simulink model "Intergration_simu"  (R2018b)
settings: Solver=FixedStepDiscrete  StartTime=0.0  StopTime=14  FixedStep=0.005  RelTol=1e-3
PostLoadFcn:
  | if any(exist('dsrtsu_mdlpostloadfcn', 'file') ~= 0), dsrtsu_mdlpostloadfcn('Execute', bdroot); end
values from neighbouring files (symbols this model uses):
  P_x165_On = 1.0    [CAN_Tx.sldd]
  P_x242_On = 1.0    [CAN_Tx.sldd]
  P_x246_On = 1.0    [CAN_Tx.sldd]
libraries: rtican x112, simulink x59
(part 31 of 31)

== system Intergration_simu/TX/ESC_FrontWheelSpeedKPH_0x123/Subsystem ==
  <WhlGndVelLDrvn_Radar> : Inport
  Bitwise Operator1 : simulink/Logic and Bit Operations/Bitwise Operator  logicop=AND  UseBitMask=on  BitMask=bin2dec('11111111')  BitMaskRealWorld=Stored Integer
  Constant : Constant  Value=0.05625
  Constant1 : Constant  Value=0.05625
  Data Type Conversion1 : DataTypeConversion  OutDataTypeStr=uint16
  Data Type Conversion2 : DataTypeConversion  OutDataTypeStr=uint8
  Divide : Product  Inputs=*/
  Multiply : Product
  Shift Arithmetic1 : ArithShift  BitShiftNumber=5  BitShiftDirection=Right
  Out1 : Outport
  Byte0 : Outport  Port=2
  Output : Outport  Port=3
  wires:
  Bitwise Operator1/1 -> Data Type Conversion2/1
  Shift Arithmetic1/1 -> Bitwise Operator1/1
  Divide/1 -> Data Type Conversion1/1
  Constant/1 -> Divide/2
  Constant1/1 -> Multiply/1
  Data Type Conversion1/1 -> Output/1, Multiply/2, Shift Arithmetic1/1
  <WhlGndVelLDrvn_Radar>/1 -> Divide/1
  Multiply/1 -> Out1/1
  Data Type Conversion2/1 -> Byte0/1

== system Intergration_simu/TX/ESC_FrontWheelSpeedKPH_0x123/Subsystem1 ==
  In1 : Inport
  <LDrvnWhlRotlDircn> : Inport  Port=2
  Add : Sum
  Bitwise Operator1 : simulink/Logic and Bit Operations/Bitwise Operator  logicop=AND  UseBitMask=on  BitMask=bin2dec('00000110')  BitMaskRealWorld=Stored Integer
  Bitwise Operator2 : simulink/Logic and Bit Operations/Bitwise Operator  logicop=AND  UseBitMask=on  BitMask=bin2dec('11111000')  BitMaskRealWorld=Stored Integer
  Data Type Conversion1 : DataTypeConversion  OutDataTypeStr=uint8
  Data Type Conversion2 : DataTypeConversion  OutDataTypeStr=uint8
  Shift Arithmetic1 : ArithShift  BitShiftNumber=1  BitShiftDirection=Left
  Shift Arithmetic2 : ArithShift  BitShiftNumber=3  BitShiftDirection=Left
  Byte1 : Outport
  wires:
  <LDrvnWhlRotlDircn>/1 -> Data Type Conversion1/1
  Bitwise Operator2/1 -> Data Type Conversion2/1
  Data Type Conversion1/1 -> Shift Arithmetic1/1
  Bitwise Operator1/1 -> Add/1
  Shift Arithmetic1/1 -> Bitwise Operator1/1
  Add/1 -> Byte1/1
  Shift Arithmetic2/1 -> Bitwise Operator2/1
  In1/1 -> Shift Arithmetic2/1
  Data Type Conversion2/1 -> Add/2

== system Intergration_simu/TX/ESC_FrontWheelSpeedKPH_0x123/Subsystem2 ==
  <WhlGndVelLDrvn_Radar> : Inport
  Bitwise Operator1 : simulink/Logic and Bit Operations/Bitwise Operator  logicop=AND  UseBitMask=on  BitMask=bin2dec('11111111')  BitMaskRealWorld=Stored Integer
  Constant : Constant  Value=0.05625
  Constant1 : Constant  Value=0.05625
  Data Type Conversion1 : DataTypeConversion  OutDataTypeStr=uint16
  Data Type Conversion2 : DataTypeConversion  OutDataTypeStr=uint8
  Divide : Product  Inputs=*/
  Multiply : Product
  Shift Arithmetic1 : ArithShift  BitShiftNumber=5  BitShiftDirection=Right
  Out1 : Outport
  Byte2 : Outport  Port=2
  Output : Outport  Port=3
  wires:
  Bitwise Operator1/1 -> Data Type Conversion2/1
  Shift Arithmetic1/1 -> Bitwise Operator1/1
  Divide/1 -> Data Type Conversion1/1
  Constant/1 -> Divide/2
  Constant1/1 -> Multiply/1
  Data Type Conversion1/1 -> Output/1, Multiply/2, Shift Arithmetic1/1
  <WhlGndVelLDrvn_Radar>/1 -> Divide/1
  Multiply/1 -> Out1/1
  Data Type Conversion2/1 -> Byte2/1

== system Intergration_simu/TX/ESC_FrontWheelSpeedKPH_0x123/Subsystem3 ==
  In1 : Inport
  <LDrvnWhlRotlDircn> : Inport  Port=2
  Add : Sum
  Bitwise Operator1 : simulink/Logic and Bit Operations/Bitwise Operator  logicop=AND  UseBitMask=on  BitMask=bin2dec('00000110')  BitMaskRealWorld=Stored Integer
  Bitwise Operator2 : simulink/Logic and Bit Operations/Bitwise Operator  logicop=AND  UseBitMask=on  BitMask=bin2dec('11111000')  BitMaskRealWorld=Stored Integer
  Data Type Conversion1 : DataTypeConversion  OutDataTypeStr=uint8
  Data Type Conversion2 : DataTypeConversion  OutDataTypeStr=uint8
  Shift Arithmetic1 : ArithShift  BitShiftNumber=1  BitShiftDirection=Left
  Shift Arithmetic2 : ArithShift  BitShiftNumber=3  BitShiftDirection=Left
  Byte3 : Outport
  wires:
  <LDrvnWhlRotlDircn>/1 -> Data Type Conversion1/1
  Bitwise Operator2/1 -> Data Type Conversion2/1
  Data Type Conversion1/1 -> Shift Arithmetic1/1
  Bitwise Operator1/1 -> Add/1
  Shift Arithmetic1/1 -> Bitwise Operator1/1
  Add/1 -> Byte3/1
  Shift Arithmetic2/1 -> Bitwise Operator2/1
  In1/1 -> Shift Arithmetic2/1
  Data Type Conversion2/1 -> Add/2

== system Intergration_simu/TX/ESC_FrontWheelSpeedKPH_0x123/Subsystem4 ==
  In1 : Inport
  Bitwise Operator2 : simulink/Logic and Bit Operations/Bitwise Operator  logicop=AND  UseBitMask=on  BitMask=bin2dec('00001111')  BitMaskRealWorld=Stored Integer
  Data Type Conversion1 : DataTypeConversion  OutDataTypeStr=uint8
  Byte6 : Outport
  wires:
  In1/1 -> Data Type Conversion1/1
  Bitwise Operator2/1 -> Byte6/1
  Data Type Conversion1/1 -> Bitwise Operator2/1

== system Intergration_simu/TX/ESC_RearWheelSpeedKPH_0x124/RollingCounter1 ==
  Add2 : Sum
  Constant5 : Constant
  Constant6 : Constant  Value=-1
  Delay : Delay  DelayLength=1
  Switch : Switch  Criteria=u2 > Threshold  Threshold=14
  RC : Outport
  wires:
  Constant6/1 -> Switch/1
  Switch/1 -> Add2/2
  Delay/1 -> RC/1, Switch/3, Switch/2
  Add2/1 -> Delay/1
  Constant5/1 -> Add2/1

== system Intergration_simu/TX/ESC_RearWheelSpeedKPH_0x124/Subsystem ==
  <WhlGndVelLDrvn_Radar> : Inport
  Bitwise Operator1 : simulink/Logic and Bit Operations/Bitwise Operator  logicop=AND  UseBitMask=on  BitMask=bin2dec('11111111')  BitMaskRealWorld=Stored Integer
  Constant : Constant  Value=0.05625
  Constant1 : Constant  Value=0.05625
  Data Type Conversion1 : DataTypeConversion  OutDataTypeStr=uint16
  Data Type Conversion2 : DataTypeConversion  OutDataTypeStr=uint8
  Divide : Product  Inputs=*/
  Multiply : Product
  Shift Arithmetic1 : ArithShift  BitShiftNumber=5  BitShiftDirection=Right
  Out1 : Outport
  Byte0 : Outport  Port=2
  Output : Outport  Port=3
  wires:
  Bitwise Operator1/1 -> Data Type Conversion2/1
  Shift Arithmetic1/1 -> Bitwise Operator1/1
  Divide/1 -> Data Type Conversion1/1
  Constant/1 -> Divide/2
  Constant1/1 -> Multiply/1
  Data Type Conversion1/1 -> Output/1, Multiply/2, Shift Arithmetic1/1
  <WhlGndVelLDrvn_Radar>/1 -> Divide/1
  Multiply/1 -> Out1/1
  Data Type Conversion2/1 -> Byte0/1

== system Intergration_simu/TX/ESC_RearWheelSpeedKPH_0x124/Subsystem1 ==
  In1 : Inport
  <LDrvnWhlRotlDircn> : Inport  Port=2
  Add : Sum
  Bitwise Operator1 : simulink/Logic and Bit Operations/Bitwise Operator  logicop=AND  UseBitMask=on  BitMask=bin2dec('00000110')  BitMaskRealWorld=Stored Integer
  Bitwise Operator2 : simulink/Logic and Bit Operations/Bitwise Operator  logicop=AND  UseBitMask=on  BitMask=bin2dec('11111000')  BitMaskRealWorld=Stored Integer
  Data Type Conversion1 : DataTypeConversion  OutDataTypeStr=uint8
  Data Type Conversion2 : DataTypeConversion  OutDataTypeStr=uint8
  Shift Arithmetic1 : ArithShift  BitShiftNumber=1  BitShiftDirection=Left
  Shift Arithmetic2 : ArithShift  BitShiftNumber=3  BitShiftDirection=Left
  Byte1 : Outport
  wires:
  <LDrvnWhlRotlDircn>/1 -> Data Type Conversion1/1
  Bitwise Operator2/1 -> Data Type Conversion2/1
  Data Type Conversion1/1 -> Shift Arithmetic1/1
  Bitwise Operator1/1 -> Add/1
  Shift Arithmetic1/1 -> Bitwise Operator1/1
  Add/1 -> Byte1/1
  Shift Arithmetic2/1 -> Bitwise Operator2/1
  In1/1 -> Shift Arithmetic2/1
  Data Type Conversion2/1 -> Add/2

== system Intergration_simu/TX/ESC_RearWheelSpeedKPH_0x124/Subsystem2 ==
  <WhlGndVelLDrvn_Radar> : Inport
  Bitwise Operator1 : simulink/Logic and Bit Operations/Bitwise Operator  logicop=AND  UseBitMask=on  BitMask=bin2dec('11111111')  BitMaskRealWorld=Stored Integer
  Constant : Constant  Value=0.05625
  Constant1 : Constant  Value=0.05625
  Data Type Conversion1 : DataTypeConversion  OutDataTypeStr=uint16
  Data Type Conversion2 : DataTypeConversion  OutDataTypeStr=uint8
  Divide : Product  Inputs=*/
  Multiply : Product
  Shift Arithmetic1 : ArithShift  BitShiftNumber=5  BitShiftDirection=Right
  Out1 : Outport
  Byte2 : Outport  Port=2
  Output : Outport  Port=3
  wires:
  Bitwise Operator1/1 -> Data Type Conversion2/1
  Shift Arithmetic1/1 -> Bitwise Operator1/1
  Divide/1 -> Data Type Conversion1/1
  Constant/1 -> Divide/2
  Constant1/1 -> Multiply/1
  Data Type Conversion1/1 -> Output/1, Multiply/2, Shift Arithmetic1/1
  <WhlGndVelLDrvn_Radar>/1 -> Divide/1
  Multiply/1 -> Out1/1
  Data Type Conversion2/1 -> Byte2/1

== system Intergration_simu/TX/ESC_RearWheelSpeedKPH_0x124/Subsystem3 ==
  In1 : Inport
  <LDrvnWhlRotlDircn> : Inport  Port=2
  Add : Sum
  Bitwise Operator1 : simulink/Logic and Bit Operations/Bitwise Operator  logicop=AND  UseBitMask=on  BitMask=bin2dec('00000110')  BitMaskRealWorld=Stored Integer
  Bitwise Operator2 : simulink/Logic and Bit Operations/Bitwise Operator  logicop=AND  UseBitMask=on  BitMask=bin2dec('11111000')  BitMaskRealWorld=Stored Integer
  Data Type Conversion1 : DataTypeConversion  OutDataTypeStr=uint8
  Data Type Conversion2 : DataTypeConversion  OutDataTypeStr=uint8
  Shift Arithmetic1 : ArithShift  BitShiftNumber=1  BitShiftDirection=Left
  Shift Arithmetic2 : ArithShift  BitShiftNumber=3  BitShiftDirection=Left
  Byte3 : Outport
  wires:
  <LDrvnWhlRotlDircn>/1 -> Data Type Conversion1/1
  Bitwise Operator2/1 -> Data Type Conversion2/1
  Data Type Conversion1/1 -> Shift Arithmetic1/1
  Bitwise Operator1/1 -> Add/1
  Shift Arithmetic1/1 -> Bitwise Operator1/1
  Add/1 -> Byte3/1
  Shift Arithmetic2/1 -> Bitwise Operator2/1
  Data Type Conversion2/1 -> Add/2
  In1/1 -> Shift Arithmetic2/1

== system Intergration_simu/TX/ESC_RearWheelSpeedKPH_0x124/Subsystem4 ==
  In1 : Inport
  Bitwise Operator2 : simulink/Logic and Bit Operations/Bitwise Operator  logicop=AND  UseBitMask=on  BitMask=bin2dec('00001111')  BitMaskRealWorld=Stored Integer
  Data Type Conversion1 : DataTypeConversion  OutDataTypeStr=uint8
  Byte6 : Outport
  wires:
  In1/1 -> Data Type Conversion1/1
  Bitwise Operator2/1 -> Byte6/1
  Data Type Conversion1/1 -> Bitwise Operator2/1

== system Intergration_simu/TX/ESC_Status_0x126/RollingCounter1 ==
  Add2 : Sum
  Constant5 : Constant
  Constant6 : Constant  Value=-1
  Delay : Delay  DelayLength=1
  Switch : Switch  Criteria=u2 > Threshold  Threshold=14
  RC : Outport
  wires:
  Constant6/1 -> Switch/1
  Switch/1 -> Add2/2
  Delay/1 -> RC/1, Switch/3, Switch/2
  Add2/1 -> Delay/1
  Constant5/1 -> Add2/1

== system Intergration_simu/TX/ESC_Status_0x126/Subsystem ==
  <WhlGndVelLDrvn_Radar> : Inport
  Bitwise Operator1 : simulink/Logic and Bit Operations/Bitwise Operator  logicop=AND  UseBitMask=on  BitMask=bin2dec('11111111')  BitMaskRealWorld=Stored Integer
  Constant : Constant  Value=0.05625
  Constant1 : Constant  Value=0.05625
  Data Type Conversion1 : DataTypeConversion  OutDataTypeStr=uint16
  Data Type Conversion2 : DataTypeConversion  OutDataTypeStr=uint8
  Divide : Product  Inputs=*/
  Multiply : Product
  Shift Arithmetic1 : ArithShift  BitShiftNumber=5  BitShiftDirection=Right
  Out1 : Outport
  Byte1 : Outport  Port=2
  Output : Outport  Port=3
  wires:
  Bitwise Operator1/1 -> Data Type Conversion2/1
  Shift Arithmetic1/1 -> Bitwise Operator1/1
  Divide/1 -> Data Type Conversion1/1
  Constant/1 -> Divide/2
  Constant1/1 -> Multiply/1
  Data Type Conversion1/1 -> Output/1, Multiply/2, Shift Arithmetic1/1
  <WhlGndVelLDrvn_Radar>/1 -> Divide/1
  Multiply/1 -> Out1/1
  Data Type Conversion2/1 -> Byte1/1

== system Intergration_simu/TX/ESC_Status_0x126/Subsystem1 ==
  In1 : Inport
  Bitwise Operator2 : simulink/Logic and Bit Operations/Bitwise Operator  logicop=AND  UseBitMask=on  BitMask=bin2dec('11111000')  BitMaskRealWorld=Stored Integer
  Data Type Conversion2 : DataTypeConversion  OutDataTypeStr=uint8
  Shift Arithmetic2 : ArithShift  BitShiftNumber=3  BitShiftDirection=Left
  Byte2 : Outport
  wires:
  In1/1 -> Shift Arithmetic2/1
  Bitwise Operator2/1 -> Data Type Conversion2/1
  Shift Arithmetic2/1 -> Bitwise Operator2/1
  Data Type Conversion2/1 -> Byte2/1

== system Intergration_simu/TX/ESC_Status_0x126/Subsystem4 ==
  In1 : Inport
  Bitwise Operator2 : simulink/Logic and Bit Operations/Bitwise Operator  logicop=AND  UseBitMask=on  BitMask=bin2dec('00001111')  BitMaskRealWorld=Stored Integer
  Data Type Conversion1 : DataTypeConversion  OutDataTypeStr=uint8
  Byte6 : Outport
  wires:
  In1/1 -> Data Type Conversion1/1
  Bitwise Operator2/1 -> Byte6/1
  Data Type Conversion1/1 -> Bitwise Operator2/1

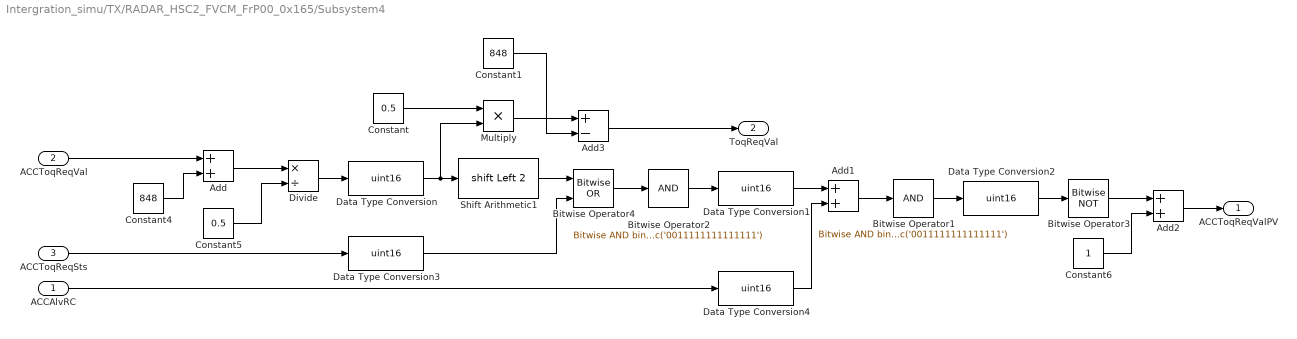
== system Intergration_simu/TX/RADAR_HSC2_FVCM_FrP00_0x165/Subsystem4 ==
  ACCAlvRC : Inport
  ACCToqReqVal : Inport  Port=2
  ACCToqReqSts : Inport  Port=3
  Add : Sum
  Add1 : Sum
  Add2 : Sum
  Add3 : Sum  Inputs=+-
  Bitwise Operator1 : simulink/Logic and Bit Operations/Bitwise Operator  logicop=AND  UseBitMask=on  BitMask=bin2dec('0011111111111111')  BitMaskRealWorld=Stored Integer
  Bitwise Operator2 : simulink/Logic and Bit Operations/Bitwise Operator  logicop=AND  UseBitMask=on  BitMask=bin2dec('0011111111111111')  BitMaskRealWorld=Stored Integer
  Bitwise Operator3 : simulink/Logic and Bit Operations/Bitwise Operator  logicop=NOT  UseBitMask=off  BitMask=bin2dec('0011111111111111')  BitMaskRealWorld=Stored Integer
  Bitwise Operator4 : simulink/Logic and Bit Operations/Bitwise Operator  logicop=OR  UseBitMask=off  NumInputPorts=2  BitMask=bin2dec('0011111111111111')  BitMaskRealWorld=Stored Integer
  Constant : Constant  Value=0.5
  Constant1 : Constant  Value=848
  Constant4 : Constant  Value=848
  Constant5 : Constant  Value=0.5
  Constant6 : Constant  OutDataTypeStr=uint16
  Data Type Conversion{,1..4} (5 alike) : DataTypeConversion  OutDataTypeStr=uint16
  Divide : Product  Inputs=*/
  Multiply : Product
  Shift Arithmetic1 : ArithShift  BitShiftNumber=2  BitShiftDirection=Left
  ACCToqReqValPV : Outport
  ToqReqVal : Outport  Port=2
  wires:
  Constant5/1 -> Divide/2
  Add/1 -> Divide/1
  Constant4/1 -> Add/2
  Data Type Conversion1/1 -> Add1/1
  Constant6/1 -> Add2/2
  Data Type Conversion/1 -> Multiply/2, Shift Arithmetic1/1
  Bitwise Operator2/1 -> Data Type Conversion1/1
  Bitwise Operator3/1 -> Add2/1
  Divide/1 -> Data Type Conversion/1
  Bitwise Operator4/1 -> Bitwise Operator2/1
  Bitwise Operator1/1 -> Data Type Conversion2/1
  Data Type Conversion2/1 -> Bitwise Operator3/1
  Shift Arithmetic1/1 -> Bitwise Operator4/1
  ACCToqReqVal/1 -> Add/1
  Add1/1 -> Bitwise Operator1/1
  ACCAlvRC/1 -> Data Type Conversion4/1
  Add2/1 -> ACCToqReqValPV/1
  ACCToqReqSts/1 -> Data Type Conversion3/1
  Data Type Conversion3/1 -> Bitwise Operator4/2
  Data Type Conversion4/1 -> Add1/2
  Constant/1 -> Multiply/1
  Multiply/1 -> Add3/1
  Constant1/1 -> Add3/2
  Add3/1 -> ToqReqVal/1

== system Intergration_simu/TX/RADAR_HSC2_FrP00_0x242/Subsystem ==
  ACCAccReqVal : Inport
  ACCSysAlvRlngCtr : Inport  Port=2
  Add : Sum
  Add1 : Sum
  Add2 : Sum  Inputs=+-
  Bitwise Operator : simulink/Logic and Bit Operations/Bitwise Operator  logicop=AND  UseBitMask=on  BitMask=bin2dec('11111111')  BitMaskRealWorld=Stored Integer
  Bitwise Operator1 : simulink/Logic and Bit Operations/Bitwise Operator  logicop=AND  UseBitMask=on  BitMask=bin2dec('00000111')  BitMaskRealWorld=Stored Integer
  Bitwise Operator2 : simulink/Logic and Bit Operations/Bitwise Operator  logicop=AND  UseBitMask=on  BitMask=bin2dec('01111000')  BitMaskRealWorld=Stored Integer
  Constant : Constant  Value=0.005
  Constant1 : Constant  Value=7.22
  Constant2 : Constant  Value=7.22
  Constant3 : Constant  Value=0.005
  Data Type Conversion : DataTypeConversion  OutDataTypeStr=uint16
  Data Type Conversion1 : DataTypeConversion  OutDataTypeStr=uint16
  Data Type Conversion2 : DataTypeConversion  OutDataTypeStr=uint8
  Data Type Conversion3 : DataTypeConversion  OutDataTypeStr=uint8
  Data Type Conversion4 : DataTypeConversion  OutDataTypeStr=uint8
  Divide : Product  Inputs=*/
  Multiply : Product
  Shift Arithmetic1 : ArithShift  BitShiftNumber=8  BitShiftDirection=Right
  Shift Arithmetic2 : ArithShift  BitShiftNumber=3  BitShiftDirection=Left
  x242_byte0 : Outport
  x242_byte1 : Outport  Port=2
  AccReqVal : Outport  Port=3
  wires:
  ACCAccReqVal/1 -> Add/1
  Data Type Conversion/1 -> Multiply/1, Bitwise Operator/1
  Divide/1 -> Data Type Conversion1/1, Data Type Conversion/1
  Bitwise Operator/1 -> Data Type Conversion4/1
  Constant2/1 -> Add/2
  Add/1 -> Divide/1
  Constant3/1 -> Divide/2
  Data Type Conversion2/1 -> Shift Arithmetic2/1
  Bitwise Operator2/1 -> Add1/1
  Bitwise Operator1/1 -> Add1/2
  Add1/1 -> x242_byte0/1
  Shift Arithmetic2/1 -> Bitwise Operator2/1
  ACCSysAlvRlngCtr/1 -> Data Type Conversion2/1
  Data Type Conversion1/1 -> Shift Arithmetic1/1
  Shift Arithmetic1/1 -> Data Type Conversion3/1
  Constant/1 -> Multiply/2
  Multiply/1 -> Add2/1
  Constant1/1 -> Add2/2
  Add2/1 -> AccReqVal/1
  Data Type Conversion3/1 -> Bitwise Operator1/1
  Data Type Conversion4/1 -> x242_byte1/1

== system Intergration_simu/TX/RADAR_HSC2_FrP00_0x242/Subsystem1 ==
  ACCAccReqSts : Inport
  ACCGoReq : Inport  Port=2
  Add : Sum
  Bitwise Operator : simulink/Logic and Bit Operations/Bitwise Operator  logicop=AND  UseBitMask=on  BitMask=bin2dec('01000000')  BitMaskRealWorld=Stored Integer
  Bitwise Operator1 : simulink/Logic and Bit Operations/Bitwise Operator  logicop=AND  UseBitMask=on  BitMask=bin2dec('00110000')  BitMaskRealWorld=Stored Integer
  Data Type Conversion1 : DataTypeConversion  OutDataTypeStr=uint8
  Data Type Conversion2 : DataTypeConversion  OutDataTypeStr=uint8
  Shift Arithmetic1 : ArithShift  BitShiftNumber=6  BitShiftDirection=Left
  Shift Arithmetic2 : ArithShift  BitShiftNumber=4  BitShiftDirection=Left
  x242_byte3 : Outport
  wires:
  Add/1 -> x242_byte3/1
  Bitwise Operator1/1 -> Add/2
  Bitwise Operator/1 -> Add/1
  Data Type Conversion1/1 -> Shift Arithmetic1/1
  Shift Arithmetic1/1 -> Bitwise Operator/1
  ACCGoReq/1 -> Data Type Conversion1/1
  Data Type Conversion2/1 -> Shift Arithmetic2/1
  Shift Arithmetic2/1 -> Bitwise Operator1/1
  ACCAccReqSts/1 -> Data Type Conversion2/1

== system Intergration_simu/TX/RADAR_HSC2_FrP00_0x242/Subsystem2 ==
  ACCSysFltSts : Inport
  ACCSysSts_Radar : Inport  Port=2
  Add : Sum
  Bitwise Operator : simulink/Logic and Bit Operations/Bitwise Operator  logicop=AND  UseBitMask=on  BitMask=bin2dec('00111000')  BitMaskRealWorld=Stored Integer
  Bitwise Operator1 : simulink/Logic and Bit Operations/Bitwise Operator  logicop=AND  UseBitMask=on  BitMask=bin2dec('00000111')  BitMaskRealWorld=Stored Integer
  Data Type Conversion1 : DataTypeConversion  OutDataTypeStr=uint8
  Data Type Conversion2 : DataTypeConversion  OutDataTypeStr=uint8
  Shift Arithmetic1 : ArithShift  BitShiftNumber=3  BitShiftDirection=Left
  x242_byte5 : Outport
  wires:
  ACCSysFltSts/1 -> Data Type Conversion2/1
  Data Type Conversion2/1 -> Bitwise Operator1/1
  Bitwise Operator/1 -> Add/1
  Add/1 -> x242_byte5/1
  Bitwise Operator1/1 -> Add/2
  Data Type Conversion1/1 -> Shift Arithmetic1/1
  Shift Arithmetic1/1 -> Bitwise Operator/1
  ACCSysSts_Radar/1 -> Data Type Conversion1/1

== system Intergration_simu/TX/RADAR_HSC2_FrP00_0x242/Subsystem3 ==
  ACCSdslReq_Radar : Inport
  Bitwise Operator2 : simulink/Logic and Bit Operations/Bitwise Operator  logicop=AND  UseBitMask=on  BitMask=bin2dec('10000000')  BitMaskRealWorld=Stored Integer
  Data Type Conversion2 : DataTypeConversion  OutDataTypeStr=uint8
  Shift Arithmetic1 : ArithShift  BitShiftNumber=7  BitShiftDirection=Left
  x242_byte6 : Outport
  wires:
  Bitwise Operator2/1 -> x242_byte6/1
  Shift Arithmetic1/1 -> Bitwise Operator2/1
  Data Type Conversion2/1 -> Shift Arithmetic1/1
  ACCSdslReq_Radar/1 -> Data Type Conversion2/1

== system Intergration_simu/TX/RADAR_HSC2_FrP01_0x244/Subsystem10 ==
  AEBSysFltSts : Inport
  Bitwise Operator3 : simulink/Logic and Bit Operations/Bitwise Operator  logicop=AND  UseBitMask=on  BitMask=bin2dec('11100000')  BitMaskRealWorld=Stored Integer
  Data Type Conversion3 : DataTypeConversion  OutDataTypeStr=uint8
  Shift Arithmetic2 : ArithShift  BitShiftNumber=5  BitShiftDirection=Left
  x244_byte5 : Outport
  wires:
  AEBSysFltSts/1 -> Data Type Conversion3/1
  Shift Arithmetic2/1 -> Bitwise Operator3/1
  Data Type Conversion3/1 -> Shift Arithmetic2/1
  Bitwise Operator3/1 -> x244_byte5/1

== system Intergration_simu/TX/RADAR_HSC2_FrP01_0x244/Subsystem5 ==
  AEBDclReqVal0 : Inport
  Add : Sum
  Add1 : Sum  Inputs=+-
  Bitwise Operator : simulink/Logic and Bit Operations/Bitwise Operator  logicop=AND  UseBitMask=on  BitMask=bin2dec('11111111')  BitMaskRealWorld=Stored Integer
  Constant : Constant  Value=12.7
  Constant1 : Constant  Value=0.1
  Constant4 : Constant  Value=0.1
  Constant5 : Constant  Value=12.7
  Data Type Conversion2 : DataTypeConversion  OutDataTypeStr=uint8
  Divide : Product  Inputs=*/  OutDataTypeStr=single
  Multiply : Product
  AEBDclReqVal : Outport
  x244_byte0 : Outport  Port=2
  wires:
  Data Type Conversion2/1 -> Bitwise Operator/1, Multiply/1
  Add/1 -> Divide/1
  Constant/1 -> Add/2
  Constant4/1 -> Multiply/2
  Divide/1 -> Data Type Conversion2/1
  Add1/1 -> AEBDclReqVal/1
  Multiply/1 -> Add1/1
  Constant5/1 -> Add1/2
  Constant1/1 -> Divide/2
  AEBDclReqVal0/1 -> Add/1
  Bitwise Operator/1 -> x244_byte0/1

== system Intergration_simu/TX/RADAR_HSC2_FrP01_0x244/Subsystem6 ==
  AEBPrflReq : Inport
  Add : Sum
  Bitwise Operator1 : simulink/Logic and Bit Operations/Bitwise Operator  logicop=AND  UseBitMask=on  BitMask=bin2dec('01111111')  BitMaskRealWorld=Stored Integer
  Bitwise Operator2 : simulink/Logic and Bit Operations/Bitwise Operator  logicop=AND  UseBitMask=on  BitMask=bin2dec('10000000')  BitMaskRealWorld=Stored Integer
  Constant : Constant  Value=0  OutDataTypeStr=uint8
  Data Type Conversion2 : DataTypeConversion  OutDataTypeStr=uint8
  Shift Arithmetic1 : ArithShift  BitShiftNumber=7  BitShiftDirection=Left
  x244_byte1 : Outport
  wires:
  Data Type Conversion2/1 -> Shift Arithmetic1/1
  Shift Arithmetic1/1 -> Bitwise Operator2/1
  AEBPrflReq/1 -> Data Type Conversion2/1
  Bitwise Operator2/1 -> Add/2
  Constant/1 -> Bitwise Operator1/1
  Add/1 -> x244_byte1/1
  Bitwise Operator1/1 -> Add/1

== system Intergration_simu/TX/RADAR_HSC2_FrP01_0x244/Subsystem7 ==
  ACCAEBBrkJerkLvlReq : Inport
  AEBSysSts : Inport  Port=2
  Add : Sum
  Bitwise Operator1 : simulink/Logic and Bit Operations/Bitwise Operator  logicop=AND  UseBitMask=on  BitMask=bin2dec('11100000')  BitMaskRealWorld=Stored Integer
  Bitwise Operator2 : simulink/Logic and Bit Operations/Bitwise Operator  logicop=AND  UseBitMask=on  BitMask=bin2dec('00011100')  BitMaskRealWorld=Stored Integer
  Data Type Conversion1 : DataTypeConversion  OutDataTypeStr=uint8
  Data Type Conversion2 : DataTypeConversion  OutDataTypeStr=uint8
  Shift Arithmetic1 : ArithShift  BitShiftNumber=2  BitShiftDirection=Left
  Shift Arithmetic2 : ArithShift  BitShiftNumber=5  BitShiftDirection=Left
  x244_byte2 : Outport
  wires:
  Shift Arithmetic1/1 -> Bitwise Operator2/1
  Shift Arithmetic2/1 -> Bitwise Operator1/1
  Add/1 -> x244_byte2/1
  AEBSysSts/1 -> Data Type Conversion1/1
  ACCAEBBrkJerkLvlReq/1 -> Data Type Conversion2/1
  Data Type Conversion2/1 -> Shift Arithmetic1/1
  Data Type Conversion1/1 -> Shift Arithmetic2/1
  Bitwise Operator2/1 -> Add/1
  Bitwise Operator1/1 -> Add/2

== system Intergration_simu/TX/RADAR_HSC2_FrP01_0x244/Subsystem8 ==
  AEBDclReqSts : Inport
  AEBPedtrnSysSts : Inport  Port=2
  AEBHydBrkAstLvlReq : Inport  Port=3
  Add : Sum  Inputs=+++
  Bitwise Operator1 : simulink/Logic and Bit Operations/Bitwise Operator  logicop=AND  UseBitMask=on  BitMask=bin2dec('00011100')  BitMaskRealWorld=Stored Integer
  Bitwise Operator2 : simulink/Logic and Bit Operations/Bitwise Operator  logicop=AND  UseBitMask=on  BitMask=bin2dec('00000011')  BitMaskRealWorld=Stored Integer
  Bitwise Operator3 : simulink/Logic and Bit Operations/Bitwise Operator  logicop=AND  UseBitMask=on  BitMask=bin2dec('11100000')  BitMaskRealWorld=Stored Integer
  Data Type Conversion1 : DataTypeConversion  OutDataTypeStr=uint8
  Data Type Conversion2 : DataTypeConversion  OutDataTypeStr=uint8
  Data Type Conversion3 : DataTypeConversion  OutDataTypeStr=uint8
  Shift Arithmetic1 : ArithShift  BitShiftNumber=2  BitShiftDirection=Left
  Shift Arithmetic2 : ArithShift  BitShiftNumber=5  BitShiftDirection=Left
  x244_byte3 : Outport
  wires:
  Bitwise Operator3/1 -> Add/1
  Shift Arithmetic1/1 -> Bitwise Operator1/1
  Bitwise Operator1/1 -> Add/3
  Data Type Conversion2/1 -> Bitwise Operator2/1
  Data Type Conversion3/1 -> Shift Arithmetic2/1
  Add/1 -> x244_byte3/1
  Shift Arithmetic2/1 -> Bitwise Operator3/1
  Bitwise Operator2/1 -> Add/2
  Data Type Conversion1/1 -> Shift Arithmetic1/1
  AEBDclReqSts/1 -> Data Type Conversion2/1
  AEBHydBrkAstLvlReq/1 -> Data Type Conversion3/1
  AEBPedtrnSysSts/1 -> Data Type Conversion1/1

== system Intergration_simu/TX/RADAR_HSC2_FrP01_0x244/Subsystem9 ==
  AEBPedtrnSysFltSts : Inport
  AEBAlvRlngCtr : Inport  Port=2
  Add : Sum
  Bitwise Operator1 : simulink/Logic and Bit Operations/Bitwise Operator  logicop=AND  UseBitMask=on  BitMask=bin2dec('00001111')  BitMaskRealWorld=Stored Integer
  Bitwise Operator3 : simulink/Logic and Bit Operations/Bitwise Operator  logicop=AND  UseBitMask=on  BitMask=bin2dec('01110000')  BitMaskRealWorld=Stored Integer
  Data Type Conversion1 : DataTypeConversion  OutDataTypeStr=uint8
  Data Type Conversion3 : DataTypeConversion  OutDataTypeStr=uint8
  Shift Arithmetic2 : ArithShift  BitShiftNumber=4  BitShiftDirection=Left
  x244_byte4 : Outport
  wires:
  Bitwise Operator1/1 -> Add/2
  Bitwise Operator3/1 -> Add/1
  Data Type Conversion1/1 -> Bitwise Operator1/1
  AEBAlvRlngCtr/1 -> Data Type Conversion1/1
  AEBPedtrnSysFltSts/1 -> Data Type Conversion3/1
  Shift Arithmetic2/1 -> Bitwise Operator3/1
  Add/1 -> x244_byte4/1
  Data Type Conversion3/1 -> Shift Arithmetic2/1

== system Intergration_simu/TX/YRS1_0x131/RollingCounter1 ==
  Add2 : Sum
  Constant5 : Constant
  Constant6 : Constant  Value=-1
  Delay : Delay  DelayLength=1
  Switch : Switch  Criteria=u2 > Threshold  Threshold=14
  RC : Outport
  wires:
  Constant6/1 -> Switch/1
  Switch/1 -> Add2/2
  Delay/1 -> RC/1, Switch/3, Switch/2
  Add2/1 -> Delay/1
  Constant5/1 -> Add2/1

== system Intergration_simu/TX/YRS1_0x131/Subsystem ==
  In1 : Inport
  Add : Sum
  Add1 : Sum  Inputs=+-
  Bitwise Operator1 : simulink/Logic and Bit Operations/Bitwise Operator  logicop=AND  UseBitMask=on  BitMask=bin2dec('11111111')  BitMaskRealWorld=Stored Integer
  Bitwise Operator2 : simulink/Logic and Bit Operations/Bitwise Operator  logicop=AND  UseBitMask=on  BitMask=bin2dec('11111111')  BitMaskRealWorld=Stored Integer
  Constant1 : Constant  Value=2
  Constant2 : Constant  Value=0.001
  Constant3 : Constant  Value=0.001
  Constant4 : Constant  Value=2
  Data Type Conversion1 : DataTypeConversion  OutDataTypeStr=uint16
  Data Type Conversion2 : DataTypeConversion  OutDataTypeStr=uint8
  Data Type Conversion3 : DataTypeConversion  OutDataTypeStr=uint8
  Divide1 : Product  Inputs=*/
  Multiply : Product
  Shift Arithmetic1 : ArithShift  BitShiftNumber=8  BitShiftDirection=Right
  Byte2 : Outport
  Out2 : Outport  Port=2
  Byte3 : Outport  Port=3
  wires:
  Constant2/1 -> Divide1/2
  Constant1/1 -> Add/2
  Data Type Conversion1/1 -> Bitwise Operator2/1, Multiply/1, Shift Arithmetic1/1
  Shift Arithmetic1/1 -> Bitwise Operator1/1
  Constant4/1 -> Add1/2
  Constant3/1 -> Multiply/2
  Multiply/1 -> Add1/1
  Bitwise Operator1/1 -> Data Type Conversion2/1
  Divide1/1 -> Data Type Conversion1/1
  Add/1 -> Divide1/1
  Add1/1 -> Out2/1
  Bitwise Operator2/1 -> Data Type Conversion3/1
  In1/1 -> Add/1
  Data Type Conversion2/1 -> Byte2/1
  Data Type Conversion3/1 -> Byte3/1

== system Intergration_simu/TX/YRS1_0x131/Subsystem1 ==
  In1 : Inport
  Add : Sum
  Add1 : Sum  Inputs=+-
  Bitwise Operator1 : simulink/Logic and Bit Operations/Bitwise Operator  logicop=AND  UseBitMask=on  BitMask=bin2dec('11111111')  BitMaskRealWorld=Stored Integer
  Bitwise Operator2 : simulink/Logic and Bit Operations/Bitwise Operator  logicop=AND  UseBitMask=on  BitMask=bin2dec('11111111')  BitMaskRealWorld=Stored Integer
  Constant1 : Constant  Value=180
  Constant2 : Constant  Value=0.01
  Constant3 : Constant  Value=0.01
  Constant4 : Constant  Value=180
  Data Type Conversion1 : DataTypeConversion  OutDataTypeStr=uint16
  Data Type Conversion2 : DataTypeConversion  OutDataTypeStr=uint8
  Data Type Conversion3 : DataTypeConversion  OutDataTypeStr=uint8
  Divide1 : Product  Inputs=*/
  Multiply : Product
  Shift Arithmetic1 : ArithShift  BitShiftNumber=8  BitShiftDirection=Right
  Byte4 : Outport
  Out2 : Outport  Port=2
  Byte5 : Outport  Port=3
  wires:
  Constant2/1 -> Divide1/2
  Constant1/1 -> Add/2
  Data Type Conversion1/1 -> Bitwise Operator2/1, Multiply/1, Shift Arithmetic1/1
  Shift Arithmetic1/1 -> Bitwise Operator1/1
  Constant4/1 -> Add1/2
  Constant3/1 -> Multiply/2
  Multiply/1 -> Add1/1
  Bitwise Operator1/1 -> Data Type Conversion3/1
  Divide1/1 -> Data Type Conversion1/1
  Add/1 -> Divide1/1
  Add1/1 -> Out2/1
  Bitwise Operator2/1 -> Data Type Conversion2/1
  In1/1 -> Add/1
  Data Type Conversion2/1 -> Byte5/1
  Data Type Conversion3/1 -> Byte4/1

== system Intergration_simu/TX/YRS1_0x131/Subsystem4 ==
  In1 : Inport
  Bitwise Operator2 : simulink/Logic and Bit Operations/Bitwise Operator  logicop=AND  UseBitMask=on  BitMask=bin2dec('00001111')  BitMaskRealWorld=Stored Integer
  Data Type Conversion1 : DataTypeConversion  OutDataTypeStr=uint8
  Byte6 : Outport
  wires:
  In1/1 -> Data Type Conversion1/1
  Bitwise Operator2/1 -> Byte6/1
  Data Type Conversion1/1 -> Bitwise Operator2/1

== system Intergration_simu/TX/YRS2_0x132/RollingCounter1 ==
  Add2 : Sum
  Constant5 : Constant
  Constant6 : Constant  Value=-1
  Delay : Delay  DelayLength=1
  Switch : Switch  Criteria=u2 > Threshold  Threshold=14
  RC : Outport
  wires:
  Constant6/1 -> Switch/1
  Switch/1 -> Add2/2
  Delay/1 -> RC/1, Switch/3, Switch/2
  Add2/1 -> Delay/1
  Constant5/1 -> Add2/1

== system Intergration_simu/TX/YRS2_0x132/Subsystem ==
  In1 : Inport
  Add : Sum
  Add1 : Sum  Inputs=+-
  Bitwise Operator1 : simulink/Logic and Bit Operations/Bitwise Operator  logicop=AND  UseBitMask=on  BitMask=bin2dec('11111111')  BitMaskRealWorld=Stored Integer
  Bitwise Operator2 : simulink/Logic and Bit Operations/Bitwise Operator  logicop=AND  UseBitMask=on  BitMask=bin2dec('11111111')  BitMaskRealWorld=Stored Integer
  Constant1 : Constant  Value=2
  Constant2 : Constant  Value=0.001
  Constant3 : Constant  Value=0.001
  Constant4 : Constant  Value=2
  Data Type Conversion1 : DataTypeConversion  OutDataTypeStr=uint16
  Data Type Conversion2 : DataTypeConversion  OutDataTypeStr=uint8
  Data Type Conversion3 : DataTypeConversion  OutDataTypeStr=uint8
  Divide1 : Product  Inputs=*/
  Multiply : Product
  Shift Arithmetic1 : ArithShift  BitShiftNumber=8  BitShiftDirection=Right
  Byte2 : Outport
  Out2 : Outport  Port=2
  Byte3 : Outport  Port=3
  wires:
  Constant2/1 -> Divide1/2
  Constant1/1 -> Add/2
  Data Type Conversion1/1 -> Bitwise Operator2/1, Multiply/1, Shift Arithmetic1/1
  Shift Arithmetic1/1 -> Bitwise Operator1/1
  Constant4/1 -> Add1/2
  Constant3/1 -> Multiply/2
  Multiply/1 -> Add1/1
  Bitwise Operator1/1 -> Data Type Conversion2/1
  Divide1/1 -> Data Type Conversion1/1
  Add/1 -> Divide1/1
  Add1/1 -> Out2/1
  Bitwise Operator2/1 -> Data Type Conversion3/1
  In1/1 -> Add/1
  Data Type Conversion2/1 -> Byte2/1
  Data Type Conversion3/1 -> Byte3/1

== system Intergration_simu/TX/YRS2_0x132/Subsystem4 ==
  In1 : Inport
  Bitwise Operator2 : simulink/Logic and Bit Operations/Bitwise Operator  logicop=AND  UseBitMask=on  BitMask=bin2dec('00001111')  BitMaskRealWorld=Stored Integer
  Data Type Conversion1 : DataTypeConversion  OutDataTypeStr=uint8
  Byte6 : Outport
  wires:
  In1/1 -> Data Type Conversion1/1
  Bitwise Operator2/1 -> Byte6/1
  Data Type Conversion1/1 -> Bitwise Operator2/1

== system Intergration_simu/RTI Data/RTI Data Store/RTI Data Store/RTI Data Store ==
  RTI Data Store : Subsystem  mask(RTI_DATA_STORE){}
      mask help:
      | RTI Data Store Block. This block is used by RTI to store internal model dependent data. Deleting this block will result in data loss.
      |
      | NEVER DELETE, COPY, OR MODIFY THIS BLOCK!
      mask Help:
      | RTI Data Store Block. This block is used by RTI to store internal model dependent data. Deleting this block will result in data loss.
      | 
      | NEVER DELETE, COPY, OR MODIFY THIS BLOCK!
      mask Display: text(0.5, 0.5, ' ', 'HorizontalAlignment', 'center');

== system Intergration_simu/RTI Data/RTI Data Store/RTI Data Store/RTI Data Store/RTI Data Store ==

== matlab function Intergration_simu/MATLAB Function1 ==
  data: fus input; target input; lane input; objdata_st input; laneData_st input; fusDet output Bus: SIMU_FUS_ST; targetDet output Bus: SIMU_TARGET_ST; laneDet output Bus: SIMU_LANEOUTPUT_ST; ATS_PO input; Egotraj input
function [fusDet,targetDet,laneDet] = fcn(fus,target, lane, objdata_st, laneData_st, ATS_PO, Egotraj)

fusDet = fus;
icnt = 0;
for i=1:40
    if (objdata_st(i).obj_information.valid == 1)   
        icnt = icnt+1;
        fusDet.Detections(icnt).Measurement(1) = objdata_st(i).obj_estimate.longPosition;
        fusDet.Detections(icnt).Measurement(2) = objdata_st(i).obj_estimate.latPosition;
        fusDet.Detections(icnt).Measurement(3) = 0;
    end        
end
fusDet.NumDetections = icnt;

targetDet = target;
if (ATS_PO.Valid == 1)
    targetDet.Detections(1).Measurement(1) = ATS_PO.dx+2.5+3.68;
    targetDet.Detections(1).Measurement(2) = ATS_PO.dy;
    targetDet.Detections(1).Measurement(3) = 0;
    targetDet.NumDetections = 1;
else
    targetDet.Detections(1).Measurement(1) = 0;
    targetDet.Detections(1).Measurement(2) = 0;
    targetDet.Detections(1).Measurement(3) = 0;
    targetDet.NumDetections = 1;
end

laneDet = lane;
if (laneData_st.leftHostLane_C0 ~= 0)
laneDet.LaneBoundaries(1).Curvature = double(2*laneData_st.leftHostLane_C2);
laneDet.LaneBoundaries(1).CurvatureDerivative = double(6*laneData_st.leftHostLane_C3);
laneDet.LaneBoundaries(1).CurveLength = 100;
laneDet.LaneBoundaries(1).HeadingAngle = double(laneData_st.leftHostLane_C1);
laneDet.LaneBoundaries(1).LateralOffset = double(laneData_st.leftHostLane_C0);
end
laneDet.LaneBoundaries(1).BoundaryType = 1;
laneDet.LaneBoundaries(1).Strength = 0.3;
laneDet.LaneBoundaries(1).Width = 0.15;

if (laneData_st.rightHostLane_C0 ~= 0)
laneDet.LaneBoundaries(2).Curvature = double(2*laneData_st.rightHostLane_C2);
laneDet.LaneBoundaries(2).CurvatureDerivative = double(6*laneData_st.rightHostLane_C3);
laneDet.LaneBoundaries(2).CurveLength = 100;
laneDet.LaneBoundaries(2).HeadingAngle = double(laneData_st.rightHostLane_C1);
laneDet.LaneBoundaries(2).LateralOffset = double(laneData_st.rightHostLane_C0);
end
laneDet.LaneBoundaries(2).BoundaryType = 1;
laneDet.LaneBoundaries(2).Strength = 0.3;
laneDet.LaneBoundaries(2).Width = 0.15;

laneDet.LaneBoundaries(3).Curvature = double(2*Egotraj.Curvature);
laneDet.LaneBoundaries(3).CurvatureDerivative = 0;
laneDet.LaneBoundaries(3).CurveLength = 100;
laneDet.LaneBoundaries(3).HeadingAngle = 0;
laneDet.LaneBoundaries(3).LateralOffset = 1.4;
laneDet.LaneBoundaries(3).BoundaryType = 2;
laneDet.LaneBoundaries(3).Strength = 0.3;
laneDet.LaneBoundaries(3).Width = 0.15;

laneDet.LaneBoundaries(4).Curvature = double(2*Egotraj.Curvature);
laneDet.LaneBoundaries(4).CurvatureDerivative = 0;
laneDet.LaneBoundaries(4).CurveLength = 100;
laneDet.LaneBoundaries(4).HeadingAngle = 0;
laneDet.LaneBoundaries(4).LateralOffset = -1.4;
laneDet.LaneBoundaries(4).BoundaryType = 2;
laneDet.LaneBoundaries(4).Strength = 0.3;
laneDet.LaneBoundaries(4).Width = 0.15;

end

== stateflow chart Intergration_simu/OutputSignal_OS ==
  settings: description=_0p0.DUMMY.222_000_
  (default) -> (junction 68)
  (junction 68) -> (junction 67) : {
      | i= i+1;
      | }
  (junction 67) -> (junction 63) [order 1] : [ i%%2== 0]
  (junction 67) -> (junction 62) [order 2]
  (junction 63) -> (junction 61) : {
      | do_10ms;
      | }
  (junction 61) -> (junction 62)
  (junction 62) -> (junction 87)
  (junction 87) -> (junction 88) [order 1] : [ i%%4==0]
  (junction 87) -> (junction 89) [order 2]
  (junction 88) -> (junction 90) : {
      | do_20ms;
      | }
  (junction 90) -> (junction 89)
  (junction 89) -> (junction 108)
  (junction 108) -> (junction 107) [order 1] : [ i>=200]
  (junction 108) -> (junction 109) [order 2]
  (junction 107) -> (junction 110) : {
      | i=0;
      | }
  (junction 110) -> (junction 109)
  data: i local int32
  events: do_20ms output FUNCTION_CALL_EVENT; do_10ms output FUNCTION_CALL_EVENT
